simulink model "HANcoder_E407_TTA_CombineModel_Membership"  (R2022a)
settings: Solver=FixedStepDiscrete  StartTime=0.0  StopTime=1  FixedStep=0.001  RelTol=1e-3
PreLoadFcn:
  | librarySetup
  | eval([bdroot,'_startup']) %Calling [modelName]_startup.m
values from neighbouring files (symbols this model uses):
  ClockOn = Simulink.Parameter    [HANcoder_E407_TTA_Chris_startup.m]    (also in HANcoder_E407_TTA_CombineModel_Membership_2022a_startup.m; HANcoder_E407_TTA_CombineModel_Membership_startup.m; HANcoder_E407_TTA_CombineModel_V2_startup.m; HANcoder_E407_TTA_CombineModel_startup.m)
  controlWidth = Simulink.Parameter    [HANcoder_E407_TTA_CombineModel_Membership_2022a_startup.m]    (also in HANcoder_E407_TTA_CombineModel_Membership_startup.m; HANcoder_E407_TTA_CombineModel_V2_startup.m)
  desiredAngle = Simulink.Parameter    [HANcoder_E407_TTA_CombineModel_Membership_2022a_startup.m]    (also in HANcoder_E407_TTA_CombineModel_Membership_startup.m; HANcoder_E407_TTA_CombineModel_V2_startup.m)
  frequency_IRQ = 1000    [HANcoder_E407_TTA_Chris_startup.m]    (also in HANcoder_E407_TTA_CombineModel_Membership_2022a_startup.m; HANcoder_E407_TTA_CombineModel_Membership_startup.m; HANcoder_E407_TTA_CombineModel_V2_startup.m; HANcoder_E407_TTA_CombineModel_startup.m)
  intVal = Simulink.Parameter    [HANcoder_E407_TTA_CombineModel_Membership_2022a_startup.m]    (also in HANcoder_E407_TTA_CombineModel_Membership_startup.m; HANcoder_E407_TTA_CombineModel_V2_startup.m)
  L0b = 1    [HANcoder_E407_KinematicAngleControl_startup.m]    (also in HANcoder_E407_TTA_CombineModel_Membership_2022a_startup.m; HANcoder_E407_TTA_CombineModel_Membership_startup.m; HANcoder_E407_TTA_CombineModel_V2_startup.m; HANcoder_E407_TTA_CombineModel_startup.m)
  L0F = 3    [HANcoder_E407_KinematicAngleControl_startup.m]    (also in HANcoder_E407_TTA_CombineModel_Membership_2022a_startup.m; HANcoder_E407_TTA_CombineModel_Membership_startup.m; HANcoder_E407_TTA_CombineModel_V2_startup.m; HANcoder_E407_TTA_CombineModel_startup.m)
  L1F = 4    [HANcoder_E407_KinematicAngleControl_startup.m]    (also in HANcoder_E407_TTA_CombineModel_Membership_2022a_startup.m; HANcoder_E407_TTA_CombineModel_Membership_startup.m; HANcoder_E407_TTA_CombineModel_V2_startup.m; HANcoder_E407_TTA_CombineModel_startup.m)
  matrixRows = Simulink.Parameter    [HANcoder_E407_TTA_Chris_startup.m]    (also in HANcoder_E407_TTA_CombineModel_Membership_2022a_startup.m; HANcoder_E407_TTA_CombineModel_Membership_startup.m; HANcoder_E407_TTA_CombineModel_V2_startup.m; HANcoder_E407_TTA_CombineModel_startup.m)
  MMBS1_ID = Simulink.Parameter    [HANcoder_E407_TTA_Chris_startup.m]    (also in HANcoder_E407_TTA_CombineModel_Membership_2022a_startup.m; HANcoder_E407_TTA_CombineModel_Membership_startup.m; HANcoder_E407_TTA_CombineModel_V2_startup.m; HANcoder_E407_TTA_CombineModel_startup.m)
  propVal = Simulink.Parameter    [HANcoder_E407_TTA_CombineModel_Membership_2022a_startup.m]    (also in HANcoder_E407_TTA_CombineModel_Membership_startup.m; HANcoder_E407_TTA_CombineModel_V2_startup.m)
  slotTime = Simulink.Parameter    [HANcoder_E407_TTA_Chris_startup.m]    (also in HANcoder_E407_TTA_CombineModel_Membership_2022a_startup.m; HANcoder_E407_TTA_CombineModel_Membership_startup.m; HANcoder_E407_TTA_CombineModel_V2_startup.m; HANcoder_E407_TTA_CombineModel_startup.m)
  SSTM1_ID = Simulink.Parameter    [HANcoder_E407_TTA_Chris_startup.m]    (also in HANcoder_E407_TTA_CombineModel_Membership_2022a_startup.m; HANcoder_E407_TTA_CombineModel_Membership_startup.m; HANcoder_E407_TTA_CombineModel_V2_startup.m; HANcoder_E407_TTA_CombineModel_startup.m)
  SYNC1_ID = Simulink.Parameter    [HANcoder_E407_TTA_Chris_startup.m]    (also in HANcoder_E407_TTA_CombineModel_Membership_2022a_startup.m; HANcoder_E407_TTA_CombineModel_Membership_startup.m; HANcoder_E407_TTA_CombineModel_V2_startup.m; HANcoder_E407_TTA_CombineModel_startup.m)
  TRCK1_ID1 = Simulink.Parameter    [HANcoder_E407_TTA_Chris_startup.m]    (also in HANcoder_E407_TTA_CombineModel_Membership_2022a_startup.m; HANcoder_E407_TTA_CombineModel_Membership_startup.m; HANcoder_E407_TTA_CombineModel_V2_startup.m; HANcoder_E407_TTA_CombineModel_startup.m)
  TRCK1_ID2 = Simulink.Parameter    [HANcoder_E407_TTA_Chris_startup.m]    (also in HANcoder_E407_TTA_CombineModel_Membership_2022a_startup.m; HANcoder_E407_TTA_CombineModel_Membership_startup.m; HANcoder_E407_TTA_CombineModel_V2_startup.m; HANcoder_E407_TTA_CombineModel_startup.m)
  TRCK1_ID3 = Simulink.Parameter    [HANcoder_E407_TTA_Chris_startup.m]    (also in HANcoder_E407_TTA_CombineModel_Membership_2022a_startup.m; HANcoder_E407_TTA_CombineModel_Membership_startup.m; HANcoder_E407_TTA_CombineModel_V2_startup.m; HANcoder_E407_TTA_CombineModel_startup.m)
  TRLS1_ID4 = Simulink.Parameter    [HANcoder_E407_TTA_Chris_startup.m]    (also in HANcoder_E407_TTA_CombineModel_Membership_2022a_startup.m; HANcoder_E407_TTA_CombineModel_Membership_startup.m; HANcoder_E407_TTA_CombineModel_V2_startup.m; HANcoder_E407_TTA_CombineModel_startup.m)
  TRLS1_ID5 = Simulink.Parameter    [HANcoder_E407_TTA_Chris_startup.m]    (also in HANcoder_E407_TTA_CombineModel_Membership_2022a_startup.m; HANcoder_E407_TTA_CombineModel_Membership_startup.m; HANcoder_E407_TTA_CombineModel_V2_startup.m; HANcoder_E407_TTA_CombineModel_startup.m)
undefined symbols (not defined in the file or in its folder): A2, A3, A4, CON2, CON3, CON4, D10, D4, D5
libraries: HANcoder_STM32_Target x20, hdlsllib x12, dspstat3 x2, simulink x1, slpidlib x1
(part 3 of 3)

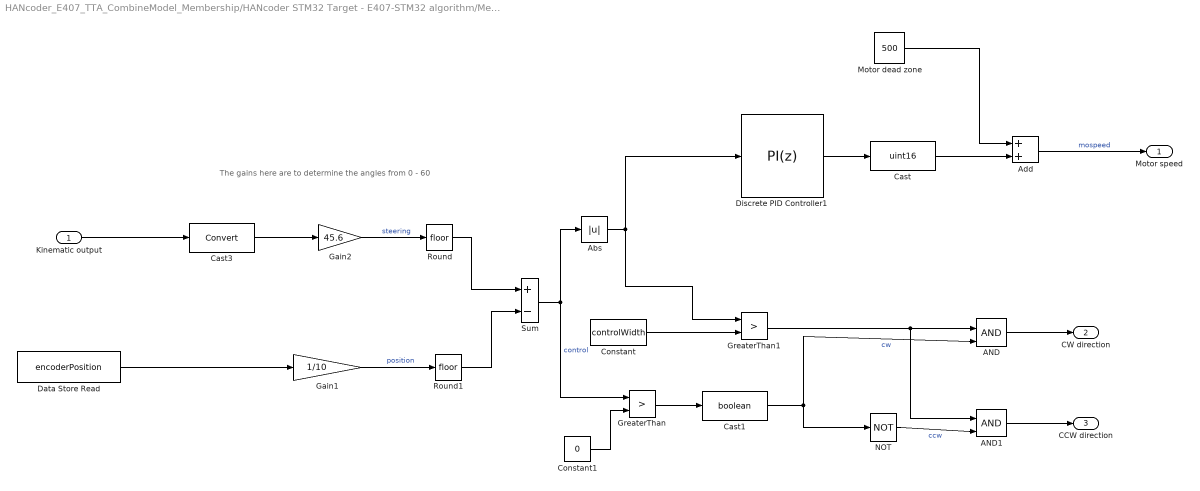
== system HANcoder_E407_TTA_CombineModel_Membership/HANcoder STM32 Target - E407-STM32 algorithm/Message selector/Subsystem/Control Algorithm ==
  note: The gains here are to determine the angles from 0 - 60
  Kinematic output : Inport
  AND : Logic  IconShape=distinctive  AllPortsSameDT=off  OutDataTypeStr=boolean
  AND1 : Logic  IconShape=distinctive  AllPortsSameDT=off  OutDataTypeStr=boolean
  Abs : Abs  OutDataTypeStr=double  SaturateOnIntegerOverflow=off
  Add : Sum  AccumDataTypeStr=uint16
  Cast : DataTypeConversion  OutDataTypeStr=uint16  SaturateOnIntegerOverflow=off  RndMeth=Floor
  Cast1 : DataTypeConversion  OutDataTypeStr=boolean  SaturateOnIntegerOverflow=off  RndMeth=Floor
  Cast3 : DataTypeConversion  SaturateOnIntegerOverflow=off  RndMeth=Floor
  Constant : Constant  Value=controlWidth
  Constant1 : Constant  Value=0
  Data Store Read : DataStoreRead  DataStoreName=encoderPosition  IndexOptions=Index vector (dialog)  Indices=1  OutputSizes=1
  Discrete PID Controller1 : slpidlib/PID Controller  Controller=PI  Form=Parallel  TimeDomain=Discrete-time  UseExternalTs=off  SampleTime=-1  IntegratorMethod=Forward Euler  FilterMethod=Forward Euler  ControllerParametersSource=internal  P=propVal  I=intVal  UseKiTs=on  D=0.5  N=100  UseFilter=on  TunerSelectOption=Transfer Function Based (PID Tuner App)  InitialConditionSource=internal  InitialConditionForIntegrator=0  InitialConditionForFilter=0  DifferentiatorICPrevScaledInput=0  ExternalReset=none  TrackingMode=off  Kt=1  LimitOutput=on  SatLimitsSource=internal  UpperSaturationLimit=300  LowerSaturationLimit=0  LinearizeAsGain=off  AntiWindupMode=clamping  Kb=1  POutMin=[]  POutMax=[]  IOutMin=[]  IOutMax=[]  DOutMin=[]  DOutMax=[]  NOutMin=[]  NOutMax=[]  SumOutMin=[]  SumOutMax=[]  SaturationOutMin=[]  SaturationOutMax=[]  PParamMin=[]  PParamMax=[]  IParamMin=[]  IParamMax=[]  DParamMin=[]  DParamMax=[]  NParamMin=[]  NParamMax=[]  KbParamMin=[]  KbParamMax=[]  KtParamMin=[]  KtParamMax=[]  KbOutMin=[]  KbOutMax=[]  KtOutMin=[]  KtOutMax=[]  IntegratorOutMin=[]  IntegratorOutMax=[]  FilterOutMin=[]  FilterOutMax=[]  SumI1OutMin=[]  SumI1OutMax=[]  SumI2OutMin=[]  SumI2OutMax=[]  SumI3OutMin=[]  SumI3OutMax=[]  SumI4OutMin=[]  SumI4OutMax=[]  SumDOutMin=[]  SumDOutMax=[]  DifferentiatorOutMin=[]  DifferentiatorOutMax=[]  FilterDiffOutCoefMin=[]  FilterDiffOutCoefMax=[]  ReciprocalOutMin=[]  ReciprocalOutMax=[]  SumDenOutMin=[]  SumDenOutMax=[]  SumNumOutMin=[]  SumNumOutMax=[]  DivideOutMin=[]  DivideOutMax=[]  UdiffTsProdOutMin=[]  UdiffTsProdOutMax=[]  NTsProdOutMin=[]  NTsProdOutMax=[]  UintegralTsProdOutMin=[]  UintegralTsProdOutMax=[]  UngainTsProdOutMin=[]  UngainTsProdOutMax=[]  IntegratorContinuousStateAttributes=''  IntegratorStateMustResolveToSignalObject=off  IntegratorRTWStateStorageClass=Auto  FilterContinuousStateAttributes=''  FilterStateMustResolveToSignalObject=off  FilterRTWStateStorageClass=Auto  ParallelPVariant=InternalParameters  IdealPVariant=Disabled  IVariant=InternalParameters  DVariant=Disabled  IntegratorVariant=Discrete  SatVariant=Enabled  AWVariant=DiscClampingParallel  PCopyVariant=Disabled  TRVariant=Disabled  FdbkBlocksVariant=Forward  IdealPFdbkVariant=Disabled  SatFdbkVariant=Disabled  DerivativeFilterVariant=Disabled  NVariant=Disabled  NCopyVariant=Disabled_SignalSpec  FilterICVariant=Disabled  IntegratorICVariant=InternalICs  ExternalResetVariant=Disabled  TRSumVariant=Passthrough  SumFdbkVariant=Disabled  SumVariant=Sum_PI  TsampFilterVariant=InternalTs  TsampNgainVariant=Passthrough  TsampIntegralVariant=Disabled_SignalSpec  ExternalSaturationOutDataTypeStr=Inherit: Same as second input
  Gain1 : Gain  Gain=1/10  OutDataTypeStr=double
  Gain2 : Gain  Gain=45.6
  GreaterThan : RelationalOperator  Operator=>  OutDataTypeStr=boolean  RndMeth=Simplest  InputSameDT=off
  GreaterThan1 : RelationalOperator  Operator=>  OutDataTypeStr=boolean  RndMeth=Simplest  InputSameDT=off
  Motor dead zone : Constant  Value=500  OutDataTypeStr=uint16
  NOT : Logic  Operator=NOT  IconShape=distinctive  AllPortsSameDT=off  OutDataTypeStr=boolean
  Round : Rounding
  Round1 : Rounding
  Sum : Sum  Inputs=+-
  Motor speed : Outport
  CW direction : Outport  Port=2
  CCW direction : Outport  Port=3
  wires:
  Motor dead zone/1 -> Add/1
  Sum/1 -> GreaterThan/1, Abs/1  "control"
  Abs/1 -> Discrete PID Controller1/1, GreaterThan1/1
  GreaterThan/1 -> Cast1/1
  Cast1/1 -> AND/2, NOT/1  "cw"
  Add/1 -> Motor speed/1  "mospeed"
  Constant1/1 -> GreaterThan/2
  Gain1/1 -> Round1/1  "position"
  Discrete PID Controller1/1 -> Cast/1
  Gain2/1 -> Round/1  "steering"
  Kinematic output/1 -> Cast3/1
  Round/1 -> Sum/1
  Round1/1 -> Sum/2
  Data Store Read/1 -> Gain1/1
  Cast3/1 -> Gain2/1
  Cast/1 -> Add/2
  GreaterThan1/1 -> AND/1, AND1/1
  Constant/1 -> GreaterThan1/2
  AND/1 -> CW direction/1
  NOT/1 -> AND1/2  "ccw"
  AND1/1 -> CCW direction/1

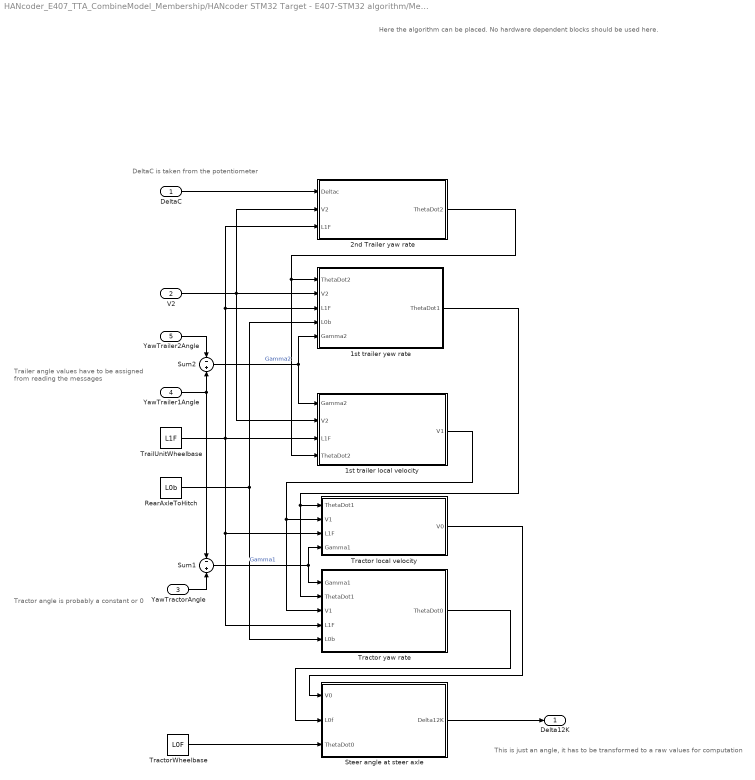
== system HANcoder_E407_TTA_CombineModel_Membership/HANcoder STM32 Target - E407-STM32 algorithm/Message selector/Subsystem/Kinematic Algorithm ==
  note: Here the algorithm can be placed. No hardware dependent blocks should be used here.
  note: Tractor angle is probably a constant or 0
  note: DeltaC is taken from the potentiometer
  note: This is just an angle, it has to be transformed to a raw values for computation
  note: Trailer angle values have to be assigned
      |  from reading the messages
  DeltaC : Inport
  V2 : Inport  Port=2
  YawTractorAngle : Inport  Port=3
  YawTrailer1Angle : Inport  Port=4
  YawTrailer2Angle : Inport  Port=5
  1st trailer local velocity : Subsystem
  1st trailer yew rate : Subsystem
  2nd Trailer yaw rate : Subsystem
  RearAxleToHitch : Constant  Value=L0b
  Steer angle at steer axle : Subsystem
  Sum1 : Sum  Inputs=-+
  Sum2 : Sum  Inputs=-+
  Tractor local velocity : Subsystem
  Tractor yaw rate : Subsystem
  TractorWheelbase : Constant  Value=L0F
  TrailUnitWheelbase : Constant  Value=L1F
  Delta12K : Outport
  wires:
  Tractor local velocity/1(V0) -> Steer angle at steer axle/1(V0)
  RearAxleToHitch/1 -> Tractor yaw rate/5(L0b), 1st trailer yew rate/4(L0b)
  2nd Trailer yaw rate/1(ThetaDot2) -> 1st trailer local velocity/4(ThetaDot2), 1st trailer yew rate/1(ThetaDot2)
  Sum2/1 -> 1st trailer local velocity/1(Gamma2), 1st trailer yew rate/5(Gamma2)  "Gamma2"
  Sum1/1 -> Tractor yaw rate/1(Gamma1), Tractor local velocity/4(Gamma1)  "Gamma1"
  1st trailer yew rate/1(ThetaDot1) -> Tractor yaw rate/2(ThetaDot1), Tractor local velocity/1(ThetaDot1)
  YawTrailer1Angle/1 -> Sum1/1, Sum2/2
  V2/1 -> 1st trailer yew rate/2(V2), 1st trailer local velocity/2(V2), 2nd Trailer yaw rate/2(V2)
  YawTrailer2Angle/1 -> Sum2/1
  TrailUnitWheelbase/1 -> Tractor yaw rate/4(L1F), Tractor local velocity/3(L1F), 1st trailer local velocity/3(L1F), 1st trailer yew rate/3(L1F), 2nd Trailer yaw rate/3(L1F)
  Steer angle at steer axle/1(Delta12K) -> Delta12K/1
  1st trailer local velocity/1(V1) -> Tractor yaw rate/3(V1), Tractor local velocity/2(V1)
  DeltaC/1 -> 2nd Trailer yaw rate/1(Deltac)
  Tractor yaw rate/1(ThetaDot0) -> Steer angle at steer axle/2(L0f)
  TractorWheelbase/1 -> Steer angle at steer axle/3(ThetaDot0)
  YawTractorAngle/1 -> Sum1/2

== system HANcoder_E407_TTA_CombineModel_Membership/HANcoder STM32 Target - E407-STM32 algorithm/Message selector/TRCK1_ID2_RX/CAN receive1 ==
  In1 : Inport
  Enabled Subsystem : Subsystem  TreatAsAtomicUnit=on
  S-Function : M-S-Function  FunctionName=sfcn_can_receive  Parameters=tsamp, canBus, outputNumber, dataType, byteOrder
  Out1 : Outport
  Out2 : Outport  Port=2
  Out3 : Outport  Port=3
  Out4 : Outport  Port=4
  Out5 : Outport  Port=5
  Out6 : Outport  Port=6
  Out7 : Outport  Port=7
  Out8 : Outport  Port=8
  Out9 : Outport  Port=9
  wires:
  S-Function/9 -> Enabled Subsystem/8(In8)
  S-Function/4 -> Enabled Subsystem/3(In3)
  S-Function/5 -> Enabled Subsystem/4(In4)
  S-Function/8 -> Enabled Subsystem/7(In7)
  S-Function/7 -> Enabled Subsystem/6(In6)
  S-Function/6 -> Enabled Subsystem/5(In5)
  Enabled Subsystem/8(Out8) -> Out9/1
  Enabled Subsystem/7(Out7) -> Out8/1
  Enabled Subsystem/6(Out6) -> Out7/1
  Enabled Subsystem/5(Out5) -> Out6/1
  Enabled Subsystem/4(Out4) -> Out5/1
  Enabled Subsystem/3(Out3) -> Out4/1
  Enabled Subsystem/2(Out2) -> Out3/1
  Enabled Subsystem/1(Out1) -> Out2/1
  S-Function/3 -> Enabled Subsystem/2(In2)
  S-Function/2 -> Enabled Subsystem/1(In1)
  S-Function/1 -> Out1/1, Enabled Subsystem/Enable
  In1/1 -> S-Function/1

== system HANcoder_E407_TTA_CombineModel_Membership/HANcoder STM32 Target - E407-STM32 algorithm/Message selector/TRCK1_ID2_TX/CAN send1 ==
  In1 : Inport
  In2 : Inport  Port=2
  In3 : Inport  Port=3
  In4 : Inport  Port=4
  In5 : Inport  Port=5
  In6 : Inport  Port=6
  Gnd7 : Ground
  Gnd8 : Ground
  Gnd9 : Ground
  S-Function : M-S-Function  FunctionName=sfcn_can_send  Parameters=tsamp, canBus, frameType, inputNumber, dataType, byteOrder
  wires:
  In1/1 -> S-Function/1
  In2/1 -> S-Function/2
  In3/1 -> S-Function/3
  In4/1 -> S-Function/4
  In5/1 -> S-Function/5
  In6/1 -> S-Function/6
  Gnd7/1 -> S-Function/7
  Gnd8/1 -> S-Function/8
  Gnd9/1 -> S-Function/9

== system HANcoder_E407_TTA_CombineModel_Membership/HANcoder STM32 Target - E407-STM32 algorithm/Message selector/TRCK1_ID2_TX/uint16to2uint1 ==
  input : Inport
  Bit Shift : hdlsllib/Logic and Bit Operations/Bit Shift  mode=Shift Right Logical  N=8
  Cast : DataTypeConversion  OutDataTypeStr=uint8  SaturateOnIntegerOverflow=off  RndMeth=Floor
  Cast1 : DataTypeConversion  OutDataTypeStr=uint8  SaturateOnIntegerOverflow=off  RndMeth=Floor
  msb : Outport
  lsb : Outport  Port=2
  wires:
  Bit Shift/1 -> Cast/1
  input/1 -> Cast1/1, Bit Shift/1
  Cast/1 -> msb/1
  Cast1/1 -> lsb/1

== system HANcoder_E407_TTA_CombineModel_Membership/HANcoder STM32 Target - E407-STM32 algorithm/Message selector/TRCK1_ID2_TX/uint16to2uint8 ==
  input : Inport
  Bit Shift : hdlsllib/Logic and Bit Operations/Bit Shift  mode=Shift Right Logical  N=8
  Cast : DataTypeConversion  OutDataTypeStr=uint8  SaturateOnIntegerOverflow=off  RndMeth=Floor
  Cast1 : DataTypeConversion  OutDataTypeStr=uint8  SaturateOnIntegerOverflow=off  RndMeth=Floor
  msb : Outport
  lsb : Outport  Port=2
  wires:
  Bit Shift/1 -> Cast/1
  input/1 -> Cast1/1, Bit Shift/1
  Cast/1 -> msb/1
  Cast1/1 -> lsb/1

== system HANcoder_E407_TTA_CombineModel_Membership/HANcoder STM32 Target - E407-STM32 algorithm/Message selector/TRCK1_ID3_TX/CAN send1 ==
  In1 : Inport
  In2 : Inport  Port=2
  In3 : Inport  Port=3
  In4 : Inport  Port=4
  In5 : Inport  Port=5
  In6 : Inport  Port=6
  Gnd7 : Ground
  Gnd8 : Ground
  Gnd9 : Ground
  S-Function : M-S-Function  FunctionName=sfcn_can_send  Parameters=tsamp, canBus, frameType, inputNumber, dataType, byteOrder
  wires:
  In1/1 -> S-Function/1
  In2/1 -> S-Function/2
  In3/1 -> S-Function/3
  In4/1 -> S-Function/4
  In5/1 -> S-Function/5
  In6/1 -> S-Function/6
  Gnd7/1 -> S-Function/7
  Gnd8/1 -> S-Function/8
  Gnd9/1 -> S-Function/9

== system HANcoder_E407_TTA_CombineModel_Membership/HANcoder STM32 Target - E407-STM32 algorithm/Message selector/TRCK1_ID3_TX/uint16to2uint1 ==
  input : Inport
  Bit Shift : hdlsllib/Logic and Bit Operations/Bit Shift  mode=Shift Right Logical  N=8
  Cast : DataTypeConversion  OutDataTypeStr=uint8  SaturateOnIntegerOverflow=off  RndMeth=Floor
  Cast1 : DataTypeConversion  OutDataTypeStr=uint8  SaturateOnIntegerOverflow=off  RndMeth=Floor
  msb : Outport
  lsb : Outport  Port=2
  wires:
  Bit Shift/1 -> Cast/1
  input/1 -> Cast1/1, Bit Shift/1
  Cast/1 -> msb/1
  Cast1/1 -> lsb/1

== system HANcoder_E407_TTA_CombineModel_Membership/HANcoder STM32 Target - E407-STM32 algorithm/Message selector/TRCK1_ID3_TX/uint16to2uint8 ==
  input : Inport
  Bit Shift : hdlsllib/Logic and Bit Operations/Bit Shift  mode=Shift Right Logical  N=8
  Cast : DataTypeConversion  OutDataTypeStr=uint8  SaturateOnIntegerOverflow=off  RndMeth=Floor
  Cast1 : DataTypeConversion  OutDataTypeStr=uint8  SaturateOnIntegerOverflow=off  RndMeth=Floor
  msb : Outport
  lsb : Outport  Port=2
  wires:
  Bit Shift/1 -> Cast/1
  input/1 -> Cast1/1, Bit Shift/1
  Cast/1 -> msb/1
  Cast1/1 -> lsb/1

== system HANcoder_E407_TTA_CombineModel_Membership/HANcoder STM32 Target - E407-STM32 algorithm/Message selector/TRCK1_RX/CAN receive1 ==
  In1 : Inport
  Enabled Subsystem : Subsystem  TreatAsAtomicUnit=on
  S-Function : M-S-Function  FunctionName=sfcn_can_receive  Parameters=tsamp, canBus, outputNumber, dataType, byteOrder
  Out1 : Outport
  Out2 : Outport  Port=2
  Out3 : Outport  Port=3
  Out4 : Outport  Port=4
  Out5 : Outport  Port=5
  Out6 : Outport  Port=6
  Out7 : Outport  Port=7
  Out8 : Outport  Port=8
  Out9 : Outport  Port=9
  wires:
  S-Function/9 -> Enabled Subsystem/8(In8)
  S-Function/4 -> Enabled Subsystem/3(In3)
  S-Function/5 -> Enabled Subsystem/4(In4)
  S-Function/8 -> Enabled Subsystem/7(In7)
  S-Function/7 -> Enabled Subsystem/6(In6)
  S-Function/6 -> Enabled Subsystem/5(In5)
  Enabled Subsystem/8(Out8) -> Out9/1
  Enabled Subsystem/7(Out7) -> Out8/1
  Enabled Subsystem/6(Out6) -> Out7/1
  Enabled Subsystem/5(Out5) -> Out6/1
  Enabled Subsystem/4(Out4) -> Out5/1
  Enabled Subsystem/3(Out3) -> Out4/1
  Enabled Subsystem/2(Out2) -> Out3/1
  Enabled Subsystem/1(Out1) -> Out2/1
  S-Function/3 -> Enabled Subsystem/2(In2)
  S-Function/2 -> Enabled Subsystem/1(In1)
  S-Function/1 -> Out1/1, Enabled Subsystem/Enable
  In1/1 -> S-Function/1

== system HANcoder_E407_TTA_CombineModel_Membership/HANcoder STM32 Target - E407-STM32 algorithm/Message selector/TRCK1_TX/CAN send1 ==
  In1 : Inport
  In2 : Inport  Port=2
  In3 : Inport  Port=3
  In4 : Inport  Port=4
  In5 : Inport  Port=5
  In6 : Inport  Port=6
  Gnd7 : Ground
  Gnd8 : Ground
  Gnd9 : Ground
  S-Function : M-S-Function  FunctionName=sfcn_can_send  Parameters=tsamp, canBus, frameType, inputNumber, dataType, byteOrder
  wires:
  In1/1 -> S-Function/1
  In2/1 -> S-Function/2
  In3/1 -> S-Function/3
  In4/1 -> S-Function/4
  In5/1 -> S-Function/5
  In6/1 -> S-Function/6
  Gnd7/1 -> S-Function/7
  Gnd8/1 -> S-Function/8
  Gnd9/1 -> S-Function/9

== system HANcoder_E407_TTA_CombineModel_Membership/HANcoder STM32 Target - E407-STM32 algorithm/Message selector/TRCK1_TX/uint16to2uint1 ==
  input : Inport
  Bit Shift : hdlsllib/Logic and Bit Operations/Bit Shift  mode=Shift Right Logical  N=8
  Cast : DataTypeConversion  OutDataTypeStr=uint8  SaturateOnIntegerOverflow=off  RndMeth=Floor
  Cast1 : DataTypeConversion  OutDataTypeStr=uint8  SaturateOnIntegerOverflow=off  RndMeth=Floor
  msb : Outport
  lsb : Outport  Port=2
  wires:
  Bit Shift/1 -> Cast/1
  input/1 -> Cast1/1, Bit Shift/1
  Cast/1 -> msb/1
  Cast1/1 -> lsb/1

== system HANcoder_E407_TTA_CombineModel_Membership/HANcoder STM32 Target - E407-STM32 algorithm/Message selector/TRCK1_TX/uint16to2uint8 ==
  input : Inport
  Bit Shift : hdlsllib/Logic and Bit Operations/Bit Shift  mode=Shift Right Logical  N=8
  Cast : DataTypeConversion  OutDataTypeStr=uint8  SaturateOnIntegerOverflow=off  RndMeth=Floor
  Cast1 : DataTypeConversion  OutDataTypeStr=uint8  SaturateOnIntegerOverflow=off  RndMeth=Floor
  msb : Outport
  lsb : Outport  Port=2
  wires:
  Bit Shift/1 -> Cast/1
  input/1 -> Cast1/1, Bit Shift/1
  Cast/1 -> msb/1
  Cast1/1 -> lsb/1

== system HANcoder_E407_TTA_CombineModel_Membership/HANcoder STM32 Target - E407-STM32 algorithm/Message selector/TRCK_ID3_RX/CAN receive1 ==
  In1 : Inport
  Enabled Subsystem : Subsystem  TreatAsAtomicUnit=on
  S-Function : M-S-Function  FunctionName=sfcn_can_receive  Parameters=tsamp, canBus, outputNumber, dataType, byteOrder
  Out1 : Outport
  Out2 : Outport  Port=2
  Out3 : Outport  Port=3
  Out4 : Outport  Port=4
  Out5 : Outport  Port=5
  Out6 : Outport  Port=6
  Out7 : Outport  Port=7
  Out8 : Outport  Port=8
  Out9 : Outport  Port=9
  wires:
  S-Function/9 -> Enabled Subsystem/8(In8)
  S-Function/4 -> Enabled Subsystem/3(In3)
  S-Function/5 -> Enabled Subsystem/4(In4)
  S-Function/8 -> Enabled Subsystem/7(In7)
  S-Function/7 -> Enabled Subsystem/6(In6)
  S-Function/6 -> Enabled Subsystem/5(In5)
  Enabled Subsystem/8(Out8) -> Out9/1
  Enabled Subsystem/7(Out7) -> Out8/1
  Enabled Subsystem/6(Out6) -> Out7/1
  Enabled Subsystem/5(Out5) -> Out6/1
  Enabled Subsystem/4(Out4) -> Out5/1
  Enabled Subsystem/3(Out3) -> Out4/1
  Enabled Subsystem/2(Out2) -> Out3/1
  Enabled Subsystem/1(Out1) -> Out2/1
  S-Function/3 -> Enabled Subsystem/2(In2)
  S-Function/2 -> Enabled Subsystem/1(In1)
  S-Function/1 -> Out1/1, Enabled Subsystem/Enable
  In1/1 -> S-Function/1

== system HANcoder_E407_TTA_CombineModel_Membership/HANcoder STM32 Target - E407-STM32 algorithm/Message selector/TRLS_ID4_RX/2bytes2uint16 ==
  MSB : Inport
  LSB : Inport  Port=2
  Add : Sum
  Bit Shift : hdlsllib/Logic and Bit Operations/Bit Shift  mode=Shift Left Logical  N=8
  Cast : DataTypeConversion  OutDataTypeStr=uint16  SaturateOnIntegerOverflow=off  RndMeth=Floor
  Cast1 : DataTypeConversion  OutDataTypeStr=uint16  SaturateOnIntegerOverflow=off  RndMeth=Floor
  uint16Out : Outport
  wires:
  Cast/1 -> Bit Shift/1
  Bit Shift/1 -> Add/1
  Cast1/1 -> Add/2
  LSB/1 -> Cast1/1
  MSB/1 -> Cast/1
  Add/1 -> uint16Out/1

== system HANcoder_E407_TTA_CombineModel_Membership/HANcoder STM32 Target - E407-STM32 algorithm/Message selector/TRLS_ID4_RX/CAN receive1 ==
  In1 : Inport
  Enabled Subsystem : Subsystem  TreatAsAtomicUnit=on
  S-Function : M-S-Function  FunctionName=sfcn_can_receive  Parameters=tsamp, canBus, outputNumber, dataType, byteOrder
  Out1 : Outport
  Out2 : Outport  Port=2
  Out3 : Outport  Port=3
  Out4 : Outport  Port=4
  Out5 : Outport  Port=5
  Out6 : Outport  Port=6
  Out7 : Outport  Port=7
  Out8 : Outport  Port=8
  Out9 : Outport  Port=9
  wires:
  S-Function/9 -> Enabled Subsystem/8(In8)
  S-Function/4 -> Enabled Subsystem/3(In3)
  S-Function/5 -> Enabled Subsystem/4(In4)
  S-Function/8 -> Enabled Subsystem/7(In7)
  S-Function/7 -> Enabled Subsystem/6(In6)
  S-Function/6 -> Enabled Subsystem/5(In5)
  Enabled Subsystem/8(Out8) -> Out9/1
  Enabled Subsystem/7(Out7) -> Out8/1
  Enabled Subsystem/6(Out6) -> Out7/1
  Enabled Subsystem/5(Out5) -> Out6/1
  Enabled Subsystem/4(Out4) -> Out5/1
  Enabled Subsystem/3(Out3) -> Out4/1
  Enabled Subsystem/2(Out2) -> Out3/1
  Enabled Subsystem/1(Out1) -> Out2/1
  S-Function/3 -> Enabled Subsystem/2(In2)
  S-Function/2 -> Enabled Subsystem/1(In1)
  S-Function/1 -> Out1/1, Enabled Subsystem/Enable
  In1/1 -> S-Function/1

== system HANcoder_E407_TTA_CombineModel_Membership/HANcoder STM32 Target - E407-STM32 algorithm/Message selector/TRLS_ID4_TX/CAN send1 ==
  In1 : Inport
  In2 : Inport  Port=2
  In3 : Inport  Port=3
  In4 : Inport  Port=4
  In5 : Inport  Port=5
  In6 : Inport  Port=6
  Gnd7 : Ground
  Gnd8 : Ground
  Gnd9 : Ground
  S-Function : M-S-Function  FunctionName=sfcn_can_send  Parameters=tsamp, canBus, frameType, inputNumber, dataType, byteOrder
  wires:
  In1/1 -> S-Function/1
  In2/1 -> S-Function/2
  In3/1 -> S-Function/3
  In4/1 -> S-Function/4
  In5/1 -> S-Function/5
  In6/1 -> S-Function/6
  Gnd7/1 -> S-Function/7
  Gnd8/1 -> S-Function/8
  Gnd9/1 -> S-Function/9

== system HANcoder_E407_TTA_CombineModel_Membership/HANcoder STM32 Target - E407-STM32 algorithm/Message selector/TRLS_ID4_TX/uint16to2uint1 ==
  input : Inport
  Bit Shift : hdlsllib/Logic and Bit Operations/Bit Shift  mode=Shift Right Logical  N=8
  Cast : DataTypeConversion  OutDataTypeStr=uint8  SaturateOnIntegerOverflow=off  RndMeth=Floor
  Cast1 : DataTypeConversion  OutDataTypeStr=uint8  SaturateOnIntegerOverflow=off  RndMeth=Floor
  msb : Outport
  lsb : Outport  Port=2
  wires:
  Bit Shift/1 -> Cast/1
  input/1 -> Cast1/1, Bit Shift/1
  Cast/1 -> msb/1
  Cast1/1 -> lsb/1

== system HANcoder_E407_TTA_CombineModel_Membership/HANcoder STM32 Target - E407-STM32 algorithm/Message selector/TRLS_ID4_TX/uint16to2uint8 ==
  input : Inport
  Bit Shift : hdlsllib/Logic and Bit Operations/Bit Shift  mode=Shift Right Logical  N=8
  Cast : DataTypeConversion  OutDataTypeStr=uint8  SaturateOnIntegerOverflow=off  RndMeth=Floor
  Cast1 : DataTypeConversion  OutDataTypeStr=uint8  SaturateOnIntegerOverflow=off  RndMeth=Floor
  msb : Outport
  lsb : Outport  Port=2
  wires:
  Bit Shift/1 -> Cast/1
  input/1 -> Cast1/1, Bit Shift/1
  Cast/1 -> msb/1
  Cast1/1 -> lsb/1

== system HANcoder_E407_TTA_CombineModel_Membership/HANcoder STM32 Target - E407-STM32 algorithm/Message selector/TRLS_ID5_RX/2bytes2uint16 ==
  MSB : Inport
  LSB : Inport  Port=2
  Add : Sum
  Bit Shift : hdlsllib/Logic and Bit Operations/Bit Shift  mode=Shift Left Logical  N=8
  Cast : DataTypeConversion  OutDataTypeStr=uint16  SaturateOnIntegerOverflow=off  RndMeth=Floor
  Cast1 : DataTypeConversion  OutDataTypeStr=uint16  SaturateOnIntegerOverflow=off  RndMeth=Floor
  uint16Out : Outport
  wires:
  Cast/1 -> Bit Shift/1
  Bit Shift/1 -> Add/1
  Cast1/1 -> Add/2
  LSB/1 -> Cast1/1
  MSB/1 -> Cast/1
  Add/1 -> uint16Out/1

== system HANcoder_E407_TTA_CombineModel_Membership/HANcoder STM32 Target - E407-STM32 algorithm/Message selector/TRLS_ID5_RX/CAN receive1 ==
  In1 : Inport
  Enabled Subsystem : Subsystem  TreatAsAtomicUnit=on
  S-Function : M-S-Function  FunctionName=sfcn_can_receive  Parameters=tsamp, canBus, outputNumber, dataType, byteOrder
  Out1 : Outport
  Out2 : Outport  Port=2
  Out3 : Outport  Port=3
  Out4 : Outport  Port=4
  Out5 : Outport  Port=5
  Out6 : Outport  Port=6
  Out7 : Outport  Port=7
  Out8 : Outport  Port=8
  Out9 : Outport  Port=9
  wires:
  S-Function/9 -> Enabled Subsystem/8(In8)
  S-Function/4 -> Enabled Subsystem/3(In3)
  S-Function/5 -> Enabled Subsystem/4(In4)
  S-Function/8 -> Enabled Subsystem/7(In7)
  S-Function/7 -> Enabled Subsystem/6(In6)
  S-Function/6 -> Enabled Subsystem/5(In5)
  Enabled Subsystem/8(Out8) -> Out9/1
  Enabled Subsystem/7(Out7) -> Out8/1
  Enabled Subsystem/6(Out6) -> Out7/1
  Enabled Subsystem/5(Out5) -> Out6/1
  Enabled Subsystem/4(Out4) -> Out5/1
  Enabled Subsystem/3(Out3) -> Out4/1
  Enabled Subsystem/2(Out2) -> Out3/1
  Enabled Subsystem/1(Out1) -> Out2/1
  S-Function/3 -> Enabled Subsystem/2(In2)
  S-Function/2 -> Enabled Subsystem/1(In1)
  S-Function/1 -> Out1/1, Enabled Subsystem/Enable
  In1/1 -> S-Function/1

== system HANcoder_E407_TTA_CombineModel_Membership/HANcoder STM32 Target - E407-STM32 algorithm/Message selector/TRLS_ID5_TX/CAN send1 ==
  In1 : Inport
  In2 : Inport  Port=2
  In3 : Inport  Port=3
  In4 : Inport  Port=4
  In5 : Inport  Port=5
  In6 : Inport  Port=6
  Gnd7 : Ground
  Gnd8 : Ground
  Gnd9 : Ground
  S-Function : M-S-Function  FunctionName=sfcn_can_send  Parameters=tsamp, canBus, frameType, inputNumber, dataType, byteOrder
  wires:
  In1/1 -> S-Function/1
  In2/1 -> S-Function/2
  In3/1 -> S-Function/3
  In4/1 -> S-Function/4
  In5/1 -> S-Function/5
  In6/1 -> S-Function/6
  Gnd7/1 -> S-Function/7
  Gnd8/1 -> S-Function/8
  Gnd9/1 -> S-Function/9

== system HANcoder_E407_TTA_CombineModel_Membership/HANcoder STM32 Target - E407-STM32 algorithm/Message selector/TRLS_ID5_TX/uint16to2uint1 ==
  input : Inport
  Bit Shift : hdlsllib/Logic and Bit Operations/Bit Shift  mode=Shift Right Logical  N=8
  Cast : DataTypeConversion  OutDataTypeStr=uint8  SaturateOnIntegerOverflow=off  RndMeth=Floor
  Cast1 : DataTypeConversion  OutDataTypeStr=uint8  SaturateOnIntegerOverflow=off  RndMeth=Floor
  msb : Outport
  lsb : Outport  Port=2
  wires:
  Bit Shift/1 -> Cast/1
  input/1 -> Cast1/1, Bit Shift/1
  Cast/1 -> msb/1
  Cast1/1 -> lsb/1

== system HANcoder_E407_TTA_CombineModel_Membership/HANcoder STM32 Target - E407-STM32 algorithm/Message selector/TRLS_ID5_TX/uint16to2uint2 ==
  input : Inport
  Bit Shift : hdlsllib/Logic and Bit Operations/Bit Shift  mode=Shift Right Logical  N=8
  Cast : DataTypeConversion  OutDataTypeStr=uint8  SaturateOnIntegerOverflow=off  RndMeth=Floor
  Cast1 : DataTypeConversion  OutDataTypeStr=uint8  SaturateOnIntegerOverflow=off  RndMeth=Floor
  msb : Outport
  lsb : Outport  Port=2
  wires:
  Bit Shift/1 -> Cast/1
  Cast/1 -> msb/1
  Cast1/1 -> lsb/1
  input/1 -> Cast1/1, Bit Shift/1

== system HANcoder_E407_TTA_CombineModel_Membership/HANcoder STM32 Target - E407-STM32 algorithm/Role assignment/Subsystem2/CAN receive1 ==
  In1 : Inport
  Enabled Subsystem : Subsystem  TreatAsAtomicUnit=on
  S-Function : M-S-Function  FunctionName=sfcn_can_receive  Parameters=tsamp, canBus, outputNumber, dataType, byteOrder
  Out1 : Outport
  Out2 : Outport  Port=2
  Out3 : Outport  Port=3
  Out4 : Outport  Port=4
  Out5 : Outport  Port=5
  Out6 : Outport  Port=6
  Out7 : Outport  Port=7
  Out8 : Outport  Port=8
  Out9 : Outport  Port=9
  wires:
  S-Function/9 -> Enabled Subsystem/8(In8)
  S-Function/4 -> Enabled Subsystem/3(In3)
  S-Function/5 -> Enabled Subsystem/4(In4)
  S-Function/8 -> Enabled Subsystem/7(In7)
  S-Function/7 -> Enabled Subsystem/6(In6)
  S-Function/6 -> Enabled Subsystem/5(In5)
  Enabled Subsystem/8(Out8) -> Out9/1
  Enabled Subsystem/7(Out7) -> Out8/1
  Enabled Subsystem/6(Out6) -> Out7/1
  Enabled Subsystem/5(Out5) -> Out6/1
  Enabled Subsystem/4(Out4) -> Out5/1
  Enabled Subsystem/3(Out3) -> Out4/1
  Enabled Subsystem/2(Out2) -> Out3/1
  Enabled Subsystem/1(Out1) -> Out2/1
  S-Function/3 -> Enabled Subsystem/2(In2)
  S-Function/2 -> Enabled Subsystem/1(In1)
  S-Function/1 -> Out1/1, Enabled Subsystem/Enable
  In1/1 -> S-Function/1

== system HANcoder_E407_TTA_CombineModel_Membership/HANcoder STM32 Target - E407-STM32 algorithm/Role assignment/Subsystem2/Subsystem1 ==
  dataArx : Inport
  Trigger : TriggerPort  VariantControl=(inherit)  PortDimensions=1
  Constant : Constant  Value=0  OutDataTypeStr=uint8
  Constant1 : Constant  OutDataTypeStr=boolean
  Constant2 : Constant  OutDataTypeStr=uint8
  Data Store Write : DataStoreWrite  DataStoreName=SlotTime  IndexOptions=Index vector (dialog)  Indices=1  OutputSizes=1
  Data Store Write1 : DataStoreWrite  DataStoreName=Local_Ticks  IndexOptions=Index vector (dialog)  Indices=1  OutputSizes=1
  Data Store Write2 : DataStoreWrite  DataStoreName=slaveClockOn  IndexOptions=Index vector (dialog)  Indices=1  OutputSizes=1
  Data Store Write3 : DataStoreWrite  DataStoreName=slot  IndexOptions=Index vector (dialog)  Indices=1  OutputSizes=1
  wires:
  dataArx/1 -> Data Store Write/1
  Constant/1 -> Data Store Write1/1
  Constant1/1 -> Data Store Write2/1
  Constant2/1 -> Data Store Write3/1

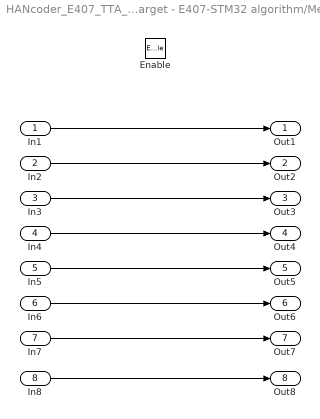
== system HANcoder_E407_TTA_CombineModel_Membership/HANcoder STM32 Target - E407-STM32 algorithm/Message selector/MMBS1_RX/CAN receive1/Enabled Subsystem ==
  In1 : Inport
  In2 : Inport  Port=2
  In3 : Inport  Port=3
  In4 : Inport  Port=4
  In5 : Inport  Port=5
  In6 : Inport  Port=6
  In7 : Inport  Port=7
  In8 : Inport  Port=8
  Enable : EnablePort
  Out1 : Outport
  Out2 : Outport  Port=2
  Out3 : Outport  Port=3
  Out4 : Outport  Port=4
  Out5 : Outport  Port=5
  Out6 : Outport  Port=6
  Out7 : Outport  Port=7
  Out8 : Outport  Port=8
  wires:
  In8/1 -> Out8/1
  In7/1 -> Out7/1
  In6/1 -> Out6/1
  In5/1 -> Out5/1
  In4/1 -> Out4/1
  In3/1 -> Out3/1
  In2/1 -> Out2/1
  In1/1 -> Out1/1

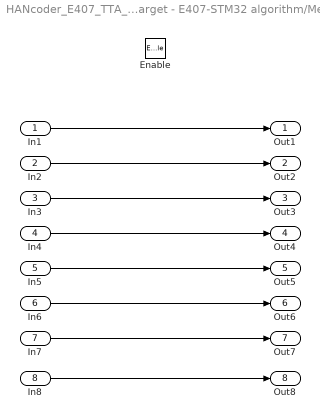
== system HANcoder_E407_TTA_CombineModel_Membership/HANcoder STM32 Target - E407-STM32 algorithm/Message selector/SSTM1_RX/CAN receive1/Enabled Subsystem ==
  In1 : Inport
  In2 : Inport  Port=2
  In3 : Inport  Port=3
  In4 : Inport  Port=4
  In5 : Inport  Port=5
  In6 : Inport  Port=6
  In7 : Inport  Port=7
  In8 : Inport  Port=8
  Enable : EnablePort
  Out1 : Outport
  Out2 : Outport  Port=2
  Out3 : Outport  Port=3
  Out4 : Outport  Port=4
  Out5 : Outport  Port=5
  Out6 : Outport  Port=6
  Out7 : Outport  Port=7
  Out8 : Outport  Port=8
  wires:
  In8/1 -> Out8/1
  In7/1 -> Out7/1
  In6/1 -> Out6/1
  In5/1 -> Out5/1
  In4/1 -> Out4/1
  In3/1 -> Out3/1
  In2/1 -> Out2/1
  In1/1 -> Out1/1

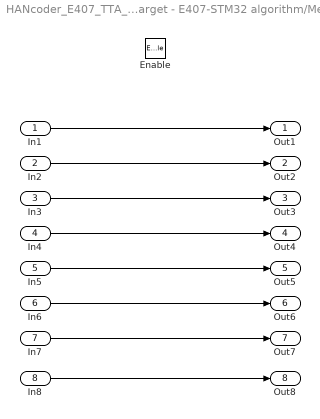
== system HANcoder_E407_TTA_CombineModel_Membership/HANcoder STM32 Target - E407-STM32 algorithm/Message selector/SYNC1_RX/CAN receive1/Enabled Subsystem ==
  In1 : Inport
  In2 : Inport  Port=2
  In3 : Inport  Port=3
  In4 : Inport  Port=4
  In5 : Inport  Port=5
  In6 : Inport  Port=6
  In7 : Inport  Port=7
  In8 : Inport  Port=8
  Enable : EnablePort
  Out1 : Outport
  Out2 : Outport  Port=2
  Out3 : Outport  Port=3
  Out4 : Outport  Port=4
  Out5 : Outport  Port=5
  Out6 : Outport  Port=6
  Out7 : Outport  Port=7
  Out8 : Outport  Port=8
  wires:
  In8/1 -> Out8/1
  In7/1 -> Out7/1
  In6/1 -> Out6/1
  In5/1 -> Out5/1
  In4/1 -> Out4/1
  In3/1 -> Out3/1
  In2/1 -> Out2/1
  In1/1 -> Out1/1

== system HANcoder_E407_TTA_CombineModel_Membership/HANcoder STM32 Target - E407-STM32 algorithm/Message selector/Slot 5 execution/Inputs/Quadrature Encoder Get ==
  Data Type Conversion : DataTypeConversion  OutDataTypeStr=boolean  SaturateOnIntegerOverflow=off  RndMeth=Floor
  Detect Increase : simulink/Logic and Bit Operations/Detect Increase  vinit=0.0  OutDataTypeStr=uint8
  Gnd1 : Ground
  Level-2 M-file S-Function : M-S-Function  FunctionName=sfcn_quad_encoder_get  Parameters=tsamp, moduleID
  Out1 : Outport
  wires:
  Level-2 M-file S-Function/1 -> Out1/1
  Gnd1/1 -> Detect Increase/1
  Detect Increase/1 -> Data Type Conversion/1
  Data Type Conversion/1 -> Level-2 M-file S-Function/1

== system HANcoder_E407_TTA_CombineModel_Membership/HANcoder STM32 Target - E407-STM32 algorithm/Message selector/Slot 5 execution/Outputs/PWM Init ==
  S-Function : S-Function  FunctionName=sfcn_pwmout_init  SFunctionDeploymentMode=off  EnableBusSupport=off
  Term1 : Terminator
  wires:
  S-Function/1 -> Term1/1

== system HANcoder_E407_TTA_CombineModel_Membership/HANcoder STM32 Target - E407-STM32 algorithm/Message selector/Subsystem/Kinematic Algorithm/1st trailer local velocity ==
  Gamma2 : Inport
  V2 : Inport  Port=2
  L1F : Inport  Port=3
  ThetaDot2 : Inport  Port=4
  Add : Sum
  Cast : DataTypeConversion  SaturateOnIntegerOverflow=off  RndMeth=Floor
  Product1 : Product  Inputs=**
  Product2 : Product  Inputs=***
  tan 1 : Trigonometry
  tan 2 : Trigonometry  Operator=cos
  V1 : Outport
  wires:
  tan 1/1 -> Product2/3
  tan 2/1 -> Product1/1
  Gamma2/1 -> Cast/1
  L1F/1 -> Product2/2
  V2/1 -> Product1/2
  Product2/1 -> Add/1  "L1f * ThetaDot2*sin(gamma2)"
  Product1/1 -> Add/2  "v2*cos(gamma2)"
  Add/1 -> V1/1
  ThetaDot2/1 -> Product2/1
  Cast/1 -> tan 1/1, tan 2/1

== system HANcoder_E407_TTA_CombineModel_Membership/HANcoder STM32 Target - E407-STM32 algorithm/Message selector/Subsystem/Kinematic Algorithm/1st trailer yew rate ==
  ThetaDot2 : Inport
  V2 : Inport  Port=2
  L1F : Inport  Port=3
  L0b : Inport  Port=4
  Gamma2 : Inport  Port=5
  Add : Sum
  Cast : DataTypeConversion  SaturateOnIntegerOverflow=off  RndMeth=Floor
  Gain : Gain  Gain=-1
  Product : Product  Inputs=***
  Product1 : Product  Inputs=*/*
  Product3 : Product  Inputs=*/**
  Sign : Signum
  Sign1 : Signum
  "tan " : Trigonometry
  tan 1 : Trigonometry  Operator=cos
  ThetaDot1 : Outport
  wires:
  V2/1 -> Product1/1, Sign/1
  L1F/1 -> Product3/3
  ThetaDot2/1 -> Product3/4
  Product3/1 -> Add/2  "(L1f/L0b)*ThetaDot2*cos(gamma2)"
  Product1/1 -> Gain/1
  Sign/1 -> Product/1  "sign(V2)"
  Gamma2/1 -> Cast/1
  Add/1 -> Product/3
  Sign1/1 -> Product/2  "sign(L0b)"
  Gain/1 -> Add/1  "-(V2/L0b*sin(gamma2)"
  Product/1 -> ThetaDot1/1
  L0b/1 -> Product1/2, Product3/2, Sign1/1
  tan 1/1 -> Product3/1
  "tan "/1 -> Product1/3
  Cast/1 -> "tan "/1, tan 1/1

== system HANcoder_E407_TTA_CombineModel_Membership/HANcoder STM32 Target - E407-STM32 algorithm/Message selector/Subsystem/Kinematic Algorithm/2nd Trailer yaw rate ==
  Deltac : Inport
  V2 : Inport  Port=2
  L1F : Inport  Port=3
  Abs : Abs  SaturateOnIntegerOverflow=off
  Product : Product  Inputs=**/
  "tan " : Trigonometry  Operator=tan
  ThetaDot2 : Outport
  wires:
  "tan "/1 -> Product/1
  Product/1 -> ThetaDot2/1
  Abs/1 -> Product/2
  V2/1 -> Abs/1
  L1F/1 -> Product/3
  Deltac/1 -> "tan "/1

== system HANcoder_E407_TTA_CombineModel_Membership/HANcoder STM32 Target - E407-STM32 algorithm/Message selector/Subsystem/Kinematic Algorithm/Steer angle at steer axle ==
  V0 : Inport
  L0f : Inport  Port=2
  ThetaDot0 : Inport  Port=3
  Cast : DataTypeConversion  SaturateOnIntegerOverflow=off  RndMeth=Floor
  Product1 : Product  Inputs=**/
  tan 1 : Trigonometry  Operator=atan
  Delta12K : Outport
  wires:
  Product1/1 -> Cast/1
  tan 1/1 -> Delta12K/1
  L0f/1 -> Product1/1
  V0/1 -> Product1/3
  ThetaDot0/1 -> Product1/2
  Cast/1 -> tan 1/1

== system HANcoder_E407_TTA_CombineModel_Membership/HANcoder STM32 Target - E407-STM32 algorithm/Message selector/Subsystem/Kinematic Algorithm/Tractor local velocity ==
  ThetaDot1 : Inport
  V1 : Inport  Port=2
  L1F : Inport  Port=3
  Gamma1 : Inport  Port=4
  Add : Sum
  Cast : DataTypeConversion  SaturateOnIntegerOverflow=off  RndMeth=Floor
  Product1 : Product  Inputs=**
  Product2 : Product  Inputs=***
  tan 1 : Trigonometry
  tan 2 : Trigonometry  Operator=cos
  V0 : Outport
  wires:
  Gamma1/1 -> Cast/1
  Product1/1 -> Add/2  "v1*cos(gamma1)"
  Product2/1 -> Add/1  "L1f * ThetaDot1*sin(gamma1)"
  Add/1 -> V0/1
  tan 2/1 -> Product1/1
  tan 1/1 -> Product2/3
  V1/1 -> Product1/2
  ThetaDot1/1 -> Product2/1
  L1F/1 -> Product2/2
  Cast/1 -> tan 1/1, tan 2/1

== system HANcoder_E407_TTA_CombineModel_Membership/HANcoder STM32 Target - E407-STM32 algorithm/Message selector/Subsystem/Kinematic Algorithm/Tractor yaw rate ==
  Gamma1 : Inport
  ThetaDot1 : Inport  Port=2
  V1 : Inport  Port=3
  L1F : Inport  Port=4
  L0b : Inport  Port=5
  Add : Sum
  Cast : DataTypeConversion  SaturateOnIntegerOverflow=off  RndMeth=Floor
  Gain : Gain  Gain=-1
  Product : Product  Inputs=***
  Product1 : Product  Inputs=*/*
  Product3 : Product  Inputs=*/**
  Sign : Signum
  Sign1 : Signum
  "tan " : Trigonometry
  tan 1 : Trigonometry  Operator=cos
  ThetaDot0 : Outport
  wires:
  V1/1 -> Product1/1, Sign/1
  L1F/1 -> Product3/3
  ThetaDot1/1 -> Product3/4
  Product3/1 -> Add/2  "(L1f/L0b)*ThetaDot1*cos(gamma1)"
  Product1/1 -> Gain/1
  Sign/1 -> Product/1  "sign(V1)"
  Gamma1/1 -> Cast/1
  Add/1 -> Product/3
  Sign1/1 -> Product/2  "sign(L0b)"
  Gain/1 -> Add/1  "-(V1/L0b*sin(gamma1)"
  Product/1 -> ThetaDot0/1
  L0b/1 -> Sign1/1, Product1/2, Product3/2
  tan 1/1 -> Product3/1
  "tan "/1 -> Product1/3
  Cast/1 -> "tan "/1, tan 1/1

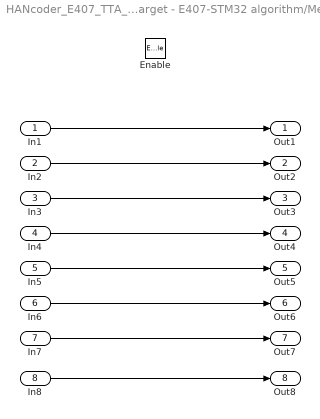
== system HANcoder_E407_TTA_CombineModel_Membership/HANcoder STM32 Target - E407-STM32 algorithm/Message selector/TRCK1_ID2_RX/CAN receive1/Enabled Subsystem ==
  In1 : Inport
  In2 : Inport  Port=2
  In3 : Inport  Port=3
  In4 : Inport  Port=4
  In5 : Inport  Port=5
  In6 : Inport  Port=6
  In7 : Inport  Port=7
  In8 : Inport  Port=8
  Enable : EnablePort
  Out1 : Outport
  Out2 : Outport  Port=2
  Out3 : Outport  Port=3
  Out4 : Outport  Port=4
  Out5 : Outport  Port=5
  Out6 : Outport  Port=6
  Out7 : Outport  Port=7
  Out8 : Outport  Port=8
  wires:
  In8/1 -> Out8/1
  In7/1 -> Out7/1
  In6/1 -> Out6/1
  In5/1 -> Out5/1
  In4/1 -> Out4/1
  In3/1 -> Out3/1
  In2/1 -> Out2/1
  In1/1 -> Out1/1

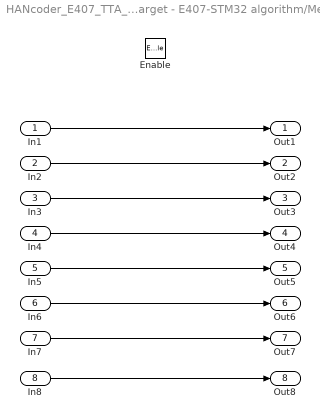
== system HANcoder_E407_TTA_CombineModel_Membership/HANcoder STM32 Target - E407-STM32 algorithm/Message selector/TRCK1_RX/CAN receive1/Enabled Subsystem ==
  In1 : Inport
  In2 : Inport  Port=2
  In3 : Inport  Port=3
  In4 : Inport  Port=4
  In5 : Inport  Port=5
  In6 : Inport  Port=6
  In7 : Inport  Port=7
  In8 : Inport  Port=8
  Enable : EnablePort
  Out1 : Outport
  Out2 : Outport  Port=2
  Out3 : Outport  Port=3
  Out4 : Outport  Port=4
  Out5 : Outport  Port=5
  Out6 : Outport  Port=6
  Out7 : Outport  Port=7
  Out8 : Outport  Port=8
  wires:
  In8/1 -> Out8/1
  In7/1 -> Out7/1
  In6/1 -> Out6/1
  In5/1 -> Out5/1
  In4/1 -> Out4/1
  In3/1 -> Out3/1
  In2/1 -> Out2/1
  In1/1 -> Out1/1

== system HANcoder_E407_TTA_CombineModel_Membership/HANcoder STM32 Target - E407-STM32 algorithm/Message selector/TRCK_ID3_RX/CAN receive1/Enabled Subsystem ==
  In1 : Inport
  In2 : Inport  Port=2
  In3 : Inport  Port=3
  In4 : Inport  Port=4
  In5 : Inport  Port=5
  In6 : Inport  Port=6
  In7 : Inport  Port=7
  In8 : Inport  Port=8
  Enable : EnablePort
  Out1 : Outport
  Out2 : Outport  Port=2
  Out3 : Outport  Port=3
  Out4 : Outport  Port=4
  Out5 : Outport  Port=5
  Out6 : Outport  Port=6
  Out7 : Outport  Port=7
  Out8 : Outport  Port=8
  wires:
  In8/1 -> Out8/1
  In7/1 -> Out7/1
  In6/1 -> Out6/1
  In5/1 -> Out5/1
  In4/1 -> Out4/1
  In3/1 -> Out3/1
  In2/1 -> Out2/1
  In1/1 -> Out1/1

== system HANcoder_E407_TTA_CombineModel_Membership/HANcoder STM32 Target - E407-STM32 algorithm/Message selector/TRLS_ID4_RX/CAN receive1/Enabled Subsystem ==
  In1 : Inport
  In2 : Inport  Port=2
  In3 : Inport  Port=3
  In4 : Inport  Port=4
  In5 : Inport  Port=5
  In6 : Inport  Port=6
  In7 : Inport  Port=7
  In8 : Inport  Port=8
  Enable : EnablePort
  Out1 : Outport
  Out2 : Outport  Port=2
  Out3 : Outport  Port=3
  Out4 : Outport  Port=4
  Out5 : Outport  Port=5
  Out6 : Outport  Port=6
  Out7 : Outport  Port=7
  Out8 : Outport  Port=8
  wires:
  In8/1 -> Out8/1
  In7/1 -> Out7/1
  In6/1 -> Out6/1
  In5/1 -> Out5/1
  In4/1 -> Out4/1
  In3/1 -> Out3/1
  In2/1 -> Out2/1
  In1/1 -> Out1/1

== system HANcoder_E407_TTA_CombineModel_Membership/HANcoder STM32 Target - E407-STM32 algorithm/Message selector/TRLS_ID5_RX/CAN receive1/Enabled Subsystem ==
  In1 : Inport
  In2 : Inport  Port=2
  In3 : Inport  Port=3
  In4 : Inport  Port=4
  In5 : Inport  Port=5
  In6 : Inport  Port=6
  In7 : Inport  Port=7
  In8 : Inport  Port=8
  Enable : EnablePort
  Out1 : Outport
  Out2 : Outport  Port=2
  Out3 : Outport  Port=3
  Out4 : Outport  Port=4
  Out5 : Outport  Port=5
  Out6 : Outport  Port=6
  Out7 : Outport  Port=7
  Out8 : Outport  Port=8
  wires:
  In8/1 -> Out8/1
  In7/1 -> Out7/1
  In6/1 -> Out6/1
  In5/1 -> Out5/1
  In4/1 -> Out4/1
  In3/1 -> Out3/1
  In2/1 -> Out2/1
  In1/1 -> Out1/1

== system HANcoder_E407_TTA_CombineModel_Membership/HANcoder STM32 Target - E407-STM32 algorithm/Role assignment/Subsystem2/CAN receive1/Enabled Subsystem ==
  In1 : Inport
  In2 : Inport  Port=2
  In3 : Inport  Port=3
  In4 : Inport  Port=4
  In5 : Inport  Port=5
  In6 : Inport  Port=6
  In7 : Inport  Port=7
  In8 : Inport  Port=8
  Enable : EnablePort
  Out1 : Outport
  Out2 : Outport  Port=2
  Out3 : Outport  Port=3
  Out4 : Outport  Port=4
  Out5 : Outport  Port=5
  Out6 : Outport  Port=6
  Out7 : Outport  Port=7
  Out8 : Outport  Port=8
  wires:
  In8/1 -> Out8/1
  In7/1 -> Out7/1
  In6/1 -> Out6/1
  In5/1 -> Out5/1
  In4/1 -> Out4/1
  In3/1 -> Out3/1
  In2/1 -> Out2/1
  In1/1 -> Out1/1
